simulink model "MARCH_v1_6"  (R2016a)
settings: Solver=FixedStepDiscrete  StartTime=0.0  StopTime=inf  FixedStep=0.001  RelTol=1e-3
InitFcn:
  | cd(fileparts(which(bdroot)));
  | 
  | init_model
  | initialize_model_testingBlocks
StartFcn:
  | cd(fileparts(which(bdroot)));
StopFcn:
  | cd(fileparts(which(bdroot)));
model workspace (MAT data in the model file):
  localValue = 1
  targetValue = 1
undefined symbols (not defined in the file or in its folder): Hip_HAA, Left_Leg, Right_Leg
libraries: xpcethercatlib x56, slrtlib x8, simulink x1, dspnetwork x1, aerolibanimutils x1
(part 1 of 2)
CloseFcn:
  | cd(fileparts(which(bdroot)));
settings Model: SimulationMode=external  Creator=Projectmarch  LastModifiedBy=Projectmarch
settings SolverCC: EnableConcurrentExecution=on
settings DataIOCC: SaveFormat=StructureWithTime
settings OptimizationCC: BlockReduction=off  OptimizeBlockIOStorage=off  BufferReuse=off  GlobalBufferReuse=off  ExpressionFolding=off  LocalBlockOutputs=off
settings HardwareCC: ProdBitPerPointer=32  ProdLargestAtomicFloat=None  ProdWordSize=32  ProdLongLongMode=on  ProdHWDeviceType=Generic->32-bit x86 compatible
settings RTWCC: SystemTargetFile=slrt.tlc  TemplateMakefile=slrt_default_tmf  Description=Simulink Real-Time

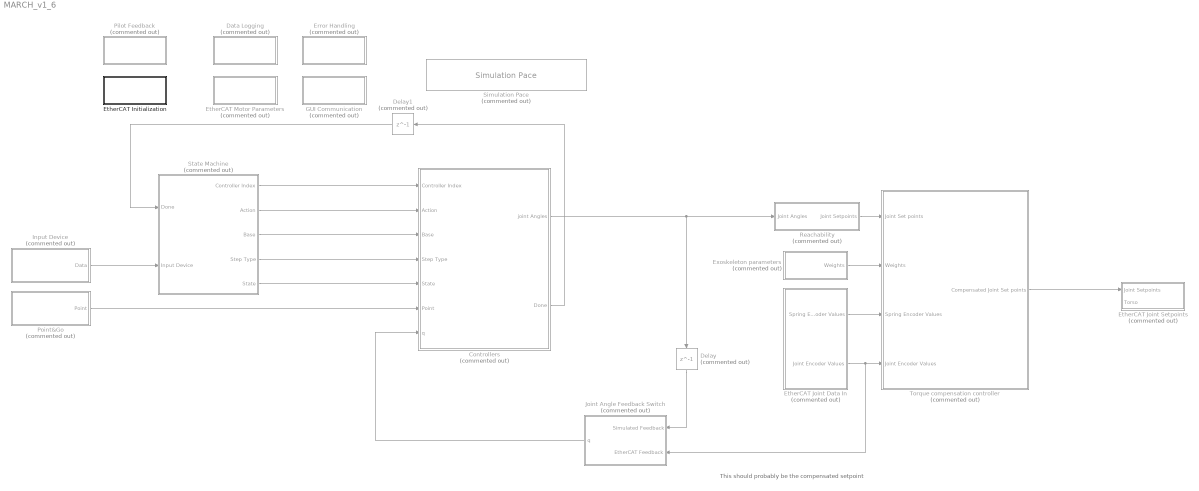
== system MARCH_v1_6 ==
  note: This should probably be the compensated setpoint
  Controllers : Subsystem  Commented=on
  Data Logging : Subsystem  Commented=on
  Delay : Delay  Commented=on  DelayLength=1
  Delay1 : Delay  Commented=on  DelayLength=1
  Error Handling : Subsystem  Commented=on
  EtherCAT Initialization : Subsystem
  EtherCAT Joint Data In : Subsystem  Commented=on
  EtherCAT Joint Setpoints : Subsystem  Commented=on
  EtherCAT Motor Parameters : Subsystem  Commented=on
  Exoskeleton parameters : Subsystem  Commented=on
  GUI Communication : Subsystem  Commented=on
  Input Device : Subsystem  Commented=on
  Joint Angle Feedback Switch : Subsystem  Commented=on
  Pilot Feedback : Subsystem  Commented=on
  Point&Go : Subsystem  Commented=on
  Reachability : Subsystem  Commented=on
  Simulation Pace : aerolibanimutils/Simulation Pace  Commented=on  SimulationPace=1  SleepMode=MATLAB Thread  OutputPaceError=off  SampleTime=-1
  State Machine : Subsystem  Commented=on
  Torque compensation controller : Subsystem  Commented=on
  wires:
  Torque compensation controller/1(Compensated Joint Set points) -> EtherCAT Joint Setpoints/1(Joint Setpoints)
  Reachability/1(Joint Setpoints) -> Torque compensation controller/1(Joint Set points)
  EtherCAT Joint Data In/1(Spring Encoder Values) -> Torque compensation controller/3(Spring Encoder Values)
  EtherCAT Joint Data In/2(Joint Encoder Values) -> Joint Angle Feedback Switch/2(EtherCAT Feedback), Torque compensation controller/4(Joint Encoder Values)
  Exoskeleton parameters/1(Weights) -> Torque compensation controller/2(Weights)
  Controllers/1(joint Angles) -> Reachability/1(Joint Angles), Delay/1
  Delay/1 -> Joint Angle Feedback Switch/1(Simulated Feedback)
  Point&Go/1(Point) -> Controllers/6(Point)
  Input Device/1(Data) -> State Machine/2(Input Device)
  Controllers/2(Done) -> Delay1/1
  State Machine/4(Step Type) -> Controllers/4(Step Type)
  State Machine/2(Action) -> Controllers/2(Action)
  State Machine/3(Base) -> Controllers/3(Base)
  State Machine/1(Controller Index) -> Controllers/1(Controller Index)
  State Machine/5(State) -> Controllers/5(State)
  Joint Angle Feedback Switch/1(q) -> Controllers/7(q)
  Delay1/1 -> State Machine/1(Done)

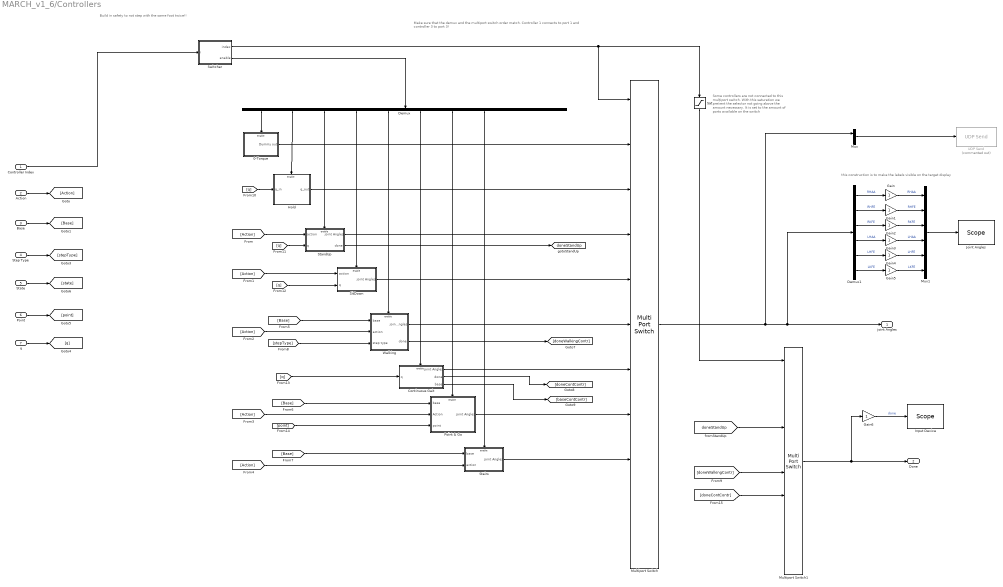
== system MARCH_v1_6/Controllers ==
  note: Some controllers are not connected to this multiport switch. With this saturation we prevent the selector not going above the amount necessary. It is set to the amount of ports available on the switch
  note: Build in safety to not step with the same
      | foot twice!!
  note: Make sure that the demux and the multiport switch order match.
      | Controller 1 connects to port 1 and controller 3 to port 3!
  note: this construction is to make the labels visible on the target display
  Controller Index : Inport
  Action : Inport  Port=2
  Base : Inport  Port=3
  Step Type : Inport  Port=4
  State : Inport  Port=5
  Point : Inport  Port=6
  q : Inport  Port=7
  0-Torque : Subsystem
  Continuous Gait : Subsystem
  Demux : Demux  Outputs=10
  Demux1 : Demux  Outputs=6
  Gain{,1..6} (7 alike) : Gain
  Hold : Subsystem
  "Input Device " : slrtlib/Displays and Logging/Scope   scopeno=4  scopetype=Target  autostart=on  viewmode=Graphical sliding  formatstr='%15.6f'  grid=on  ylimits=[0,0]  nosamples=25000  noprepostsamples=0  interleave=1  triggermode=FreeRun  triggersignal=1  trigsignalfromport=off  triggerlevel=0.0  triggerslope=Either  triggerscope=1  triggersample=0  filename=data.dat  mode=Lazy  writesize=512  autorestart=off  dynamicfilemode=off  maxwritefilesize=512*1024^2
  Joint Angles : slrtlib/Displays and Logging/Scope   scopeno=3  scopetype=Target  autostart=on  viewmode=Graphical sliding  formatstr='%15.6f'  grid=on  ylimits=[0,0]  nosamples=25000  noprepostsamples=0  interleave=1  triggermode=FreeRun  triggersignal=1  trigsignalfromport=off  triggerlevel=0.0  triggerslope=Either  triggerscope=1  triggersample=0  filename=data.dat  mode=Lazy  writesize=512  autorestart=off  dynamicfilemode=off  maxwritefilesize=512*1024^2
  Multiport Switch : MultiPortSwitch  Inputs=10
  Multiport Switch1 : MultiPortSwitch  Inputs=8  DataPortForDefault=Additional data port
  Mux : Mux  Inputs=2
  Mux1 : Mux  Inputs=6
  Point & Go : Subsystem
  Saturation : Saturate  UpperLimit=8  LowerLimit=1
  SitDown : Subsystem
  Stairs : Subsystem
  StandUp : Subsystem
  Switcher : MATLAB Function  TreatAsAtomicUnit=on
  UDP Send : dspnetwork/UDP Send  Commented=on  remoteURL='127.0.0.1'  remotePort=25000  localURL='0.0.0.0'  localPortSource=Automatically determine  localPort=-1  sampletime=-1  separateLengthPort=0
  Walking : Subsystem
  joint Angles : Outport
  Done : Outport  Port=2
  tag scope: doneStandUp=global
  wires:
  Controller Index/1 -> Switcher/1(i)
  Switcher/1(index) -> Saturation/1, Multiport Switch/1
  Switcher/2(enable) -> Demux/1
  Multiport Switch1/1 -> Gain6/1, Done/1
  Mux/1 -> UDP Send/1
  Saturation/1 -> Multiport Switch1/1
  Demux/1 -> 0-Torque/Enable
  Demux/2 -> Hold/Enable
  Demux/3 -> StandUp/Enable
  Demux/4 -> SitDown/Enable
  Demux/5 -> Walking/Enable
  Demux/6 -> Continuous Gait/Enable
  Demux/7 -> Point & Go/Enable
  Demux/8 -> Stairs/Enable
  0-Torque/1(Dummy out) -> Multiport Switch/2
  Hold/1(q_out) -> Multiport Switch/3
  StandUp/1(joint Angles) -> Multiport Switch/4
  SitDown/1(joint Angles) -> Multiport Switch/5
  Walking/1(joint Angles) -> Multiport Switch/6
  Point & Go/1(joint Angles) -> Multiport Switch/8
  Stairs/1(joint Angles) -> Multiport Switch/9
  Action/1 -> [Action]
  Base/1 -> [Base]
  Point/1 -> [point]
  q/1 -> [q]
  Step Type/1 -> [stepType]
  [Action] -> StandUp/1(action)
  [Action] -> SitDown/1(action)
  [Action] -> Walking/2(action)
  [Action] -> Point & Go/2(Action)
  [Action] -> Stairs/2(action)
  [Base] -> Walking/1(base)
  [Base] -> Point & Go/1(base)
  [Base] -> Stairs/1(base)
  [stepType] -> Walking/3(step type)
  [q] -> Hold/1(q_in)
  [q] -> StandUp/2("q ")
  [q] -> SitDown/2("q ")
  [q] -> Continuous Gait/1(q)
  [point] -> Point & Go/3(point)
  Walking/2(done) -> [doneWalkingContr]
  Continuous Gait/2(done) -> [doneContContr]
  Continuous Gait/3(base) -> [baseContContr]
  [doneWalkingContr] -> Multiport Switch1/6
  [doneContContr] -> Multiport Switch1/7
  State/1 -> [state]
  Continuous Gait/1(joint Angles) -> Multiport Switch/7
  StandUp/2(done) -> [doneStandUp]
  [doneStandUp] -> Multiport Switch1/4
  Multiport Switch/1 -> Mux/1, joint Angles/1, Demux1/1
  Demux1/1 -> Gain/1  "RHAA"
  Demux1/2 -> Gain1/1  "RHFE"
  Demux1/3 -> Gain2/1  "RKFE"
  Demux1/4 -> Gain3/1  "LHAA"
  Demux1/5 -> Gain4/1  "LHFE"
  Demux1/6 -> Gain5/1  "LKFE"
  Mux1/1 -> Joint Angles/1
  Gain/1 -> Mux1/1  "RHAA"
  Gain1/1 -> Mux1/2  "RHFE"
  Gain2/1 -> Mux1/3  "RKFE"
  Gain3/1 -> Mux1/4  "LHAA"
  Gain4/1 -> Mux1/5  "LHFE"
  Gain5/1 -> Mux1/6  "LKFE"
  Gain6/1 -> "Input Device "/1  "done"

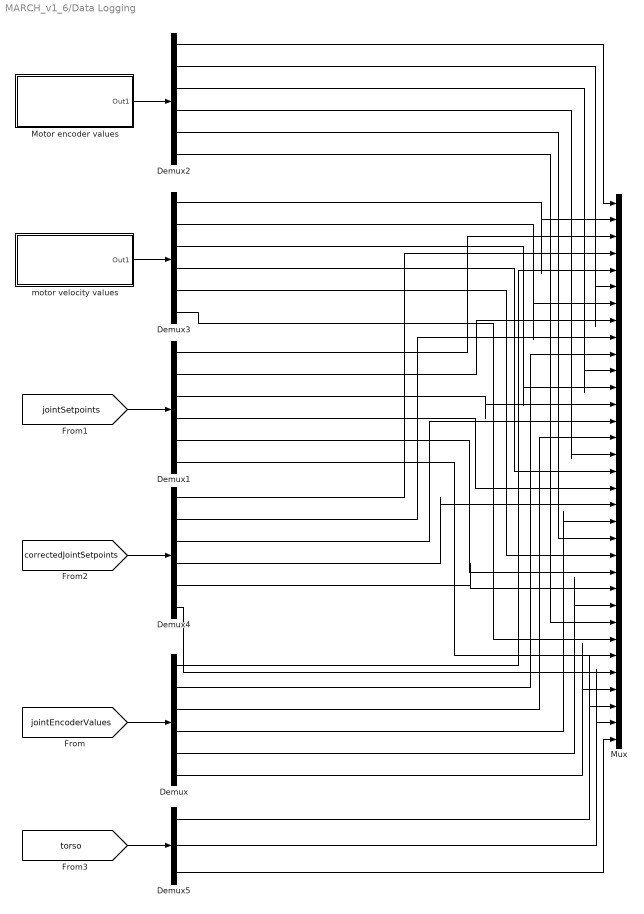
== system MARCH_v1_6/Data Logging ==
  Demux{,1..4} (5 alike) : Demux  Outputs=6
  Demux5 : Demux  Outputs=3
  Motor encoder values : Subsystem
  Mux : Mux  Inputs=33
  motor velocity values : Subsystem
  wires:
  [jointEncoderValues] -> Demux/1
  [jointSetpoints] -> Demux1/1
  Motor encoder values/1(Out1) -> Demux2/1
  motor velocity values/1(Out1) -> Demux3/1
  Demux2/1 -> Mux/1
  Demux3/1 -> Mux/2
  [correctedJointSetpoints] -> Demux4/1
  [torso] -> Demux5/1
  Demux1/1 -> Mux/3
  Demux4/1 -> Mux/4
  Demux/1 -> Mux/5
  Demux2/2 -> Mux/6
  Demux3/2 -> Mux/7
  Demux1/2 -> Mux/8
  Demux4/2 -> Mux/9
  Demux/2 -> Mux/10
  Demux2/3 -> Mux/11
  Demux3/3 -> Mux/12
  Demux1/3 -> Mux/13
  Demux4/3 -> Mux/14
  Demux/3 -> Mux/15
  Demux2/4 -> Mux/16
  Demux2/6 -> Mux/26
  Demux3/4 -> Mux/17
  Demux1/4 -> Mux/18
  Demux4/4 -> Mux/19
  Demux/4 -> Mux/20
  Demux2/5 -> Mux/21
  Demux3/5 -> Mux/22
  Demux1/5 -> Mux/23
  Demux4/5 -> Mux/24
  Demux/5 -> Mux/25
  Demux3/6 -> Mux/27
  Demux1/6 -> Mux/28
  Demux5/3 -> Mux/33
  Demux5/2 -> Mux/32
  Demux5/1 -> Mux/31
  Demux/6 -> Mux/30
  Demux4/6 -> Mux/29

== system MARCH_v1_6/Error Handling ==

== system MARCH_v1_6/EtherCAT Initialization ==
  EtherCAT Init : xpcethercatlib/EtherCAT Init   Priority=0  config_file=D:\Software\MATLAB\simulink-models\EtherCAT Config files\full_setup_v1.0.xml  device_id=0  pci_bus=2  pci_slot=0  dctuning=1  enaDebug=off  enaDC=on  errLink=on  masterDbg=on  stateChgDbg=on  baseClock=off  masterCfg=off  logFile='c:\dbglog.txt'  sample_time=0.001000
  Terminator : Terminator
  wires:
  EtherCAT Init/1 -> Terminator/1

== system MARCH_v1_6/EtherCAT Joint Data In ==
  Data Type Conversion : DataTypeConversion  OutDataTypeStr=double
  Joint Encoder EtherCAT : Subsystem
  MATLAB Function : MATLAB Function  TreatAsAtomicUnit=on
  Spring Encoder EtherCAT : Subsystem
  Spring Encoder Values : Outport
  Joint Encoder Values : Outport  Port=2
  tag scope: jointEncoderValues=global
  wires:
  Spring Encoder EtherCAT/1(Spring Encoder Values) -> Spring Encoder Values/1
  Joint Encoder EtherCAT/1(Joint Encoder Values) -> Data Type Conversion/1, [jointEncoderValues]
  MATLAB Function/1(angles) -> Joint Encoder Values/1
  Data Type Conversion/1 -> MATLAB Function/1(encoderValue)

== system MARCH_v1_6/EtherCAT Joint Setpoints ==
  Joint Setpoints : Inport
  Torso : Inport  Port=2
  Subsystem : Subsystem
  exoskeleton : Subsystem
  wires:
  Joint Setpoints/1 -> exoskeleton/1(Joint setpoints), Subsystem/1(Joint Setpoints)
  Torso/1 -> Subsystem/2(Torso)

== system MARCH_v1_6/EtherCAT Motor Parameters ==
  Hips : Subsystem
  Left Leg : Subsystem
  Right Leg : Subsystem

== system MARCH_v1_6/Exoskeleton parameters ==
  Constant : Constant
  Weights : Outport
  wires:
  Constant/1 -> Weights/1

== system MARCH_v1_6/GUI Communication ==

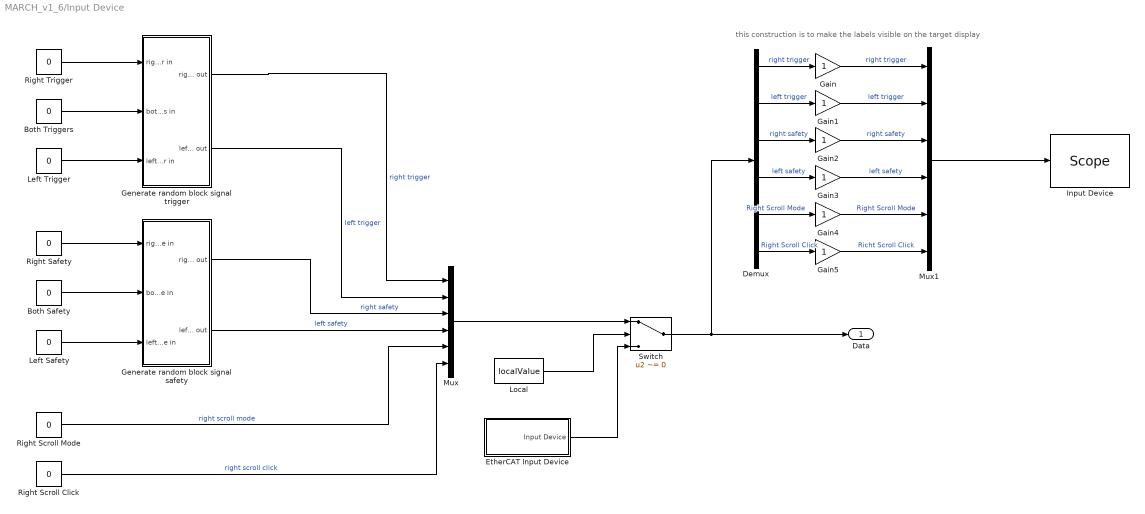
== system MARCH_v1_6/Input Device ==
  note: this construction is to make the labels visible on the target display
  Both Safety : Constant  Value=0
  Both Triggers : Constant  Value=0
  Demux : Demux  Outputs=6
  EtherCAT Input Device : Subsystem
  Gain{,1..5} (6 alike) : Gain
  Generate random block signal safety : Subsystem
  Generate random block signal trigger : Subsystem
  "Input Device " : slrtlib/Displays and Logging/Scope   scopeno=1  scopetype=Target  autostart=on  viewmode=Numerical  formatstr='%15.6f'  grid=on  ylimits=[0,0]  nosamples=25  noprepostsamples=0  interleave=1  triggermode=FreeRun  triggersignal=1  trigsignalfromport=off  triggerlevel=0.0  triggerslope=Either  triggerscope=1  triggersample=0  filename=data.dat  mode=Lazy  writesize=512  autorestart=off  dynamicfilemode=off  maxwritefilesize=512*1024^2
  Left Safety : Constant  Value=0
  Left Trigger : Constant  Value=0
  Local : Constant  Value=localValue
  Mux : Mux  Inputs=6
  Mux1 : Mux  Inputs=6
  Right Safety : Constant  Value=0
  Right Scroll Click : Constant  Value=0
  Right Scroll Mode : Constant  Value=0
  Right Trigger : Constant  Value=0
  Switch : Switch  Criteria=u2 ~= 0
  Data : Outport
  wires:
  Mux/1 -> Switch/1
  Switch/1 -> Demux/1, Data/1
  Local/1 -> Switch/2
  EtherCAT Input Device/1(Input Device) -> Switch/3
  Right Scroll Mode/1 -> Mux/5  "right scroll mode"
  Right Safety/1 -> Generate random block signal safety/1(right safe in)
  Right Scroll Click/1 -> Mux/6  "right scroll click"
  Right Trigger/1 -> Generate random block signal trigger/1(rightTrigger in)
  Left Trigger/1 -> Generate random block signal trigger/3("leftTrigger in ")
  Both Triggers/1 -> Generate random block signal trigger/2(bothTriggers in)
  Generate random block signal trigger/1(rightTrigger out) -> Mux/1  "right trigger"
  Generate random block signal trigger/2(leftTrigger out) -> Mux/2  "left trigger"
  Generate random block signal safety/1(right safe out) -> Mux/3  "right safety"
  Generate random block signal safety/2(left safe out) -> Mux/4  "left safety"
  Left Safety/1 -> Generate random block signal safety/3("left safe in ")
  Both Safety/1 -> Generate random block signal safety/2(both safe in)
  Mux1/1 -> "Input Device "/1
  Demux/1 -> Gain/1  "right trigger"
  Demux/2 -> Gain1/1  "left trigger"
  Demux/3 -> Gain2/1  "right safety"
  Demux/4 -> Gain3/1  "left safety"
  Demux/5 -> Gain4/1  "Right Scroll Mode"
  Demux/6 -> Gain5/1  "Right Scroll Click"
  Gain/1 -> Mux1/1  "right trigger"
  Gain1/1 -> Mux1/2  "left trigger"
  Gain2/1 -> Mux1/3  "right safety"
  Gain3/1 -> Mux1/4  "left safety"
  Gain4/1 -> Mux1/5  "Right Scroll Mode"
  Gain5/1 -> Mux1/6  "Richt Scroll Click"

== system MARCH_v1_6/Joint Angle Feedback Switch ==
  Simulated Feedback : Inport
  EtherCAT Feedback : Inport  Port=2
  Local : Constant  Value=0
  Switch : Switch  Criteria=u2 ~= 0
  q : Outport
  wires:
  EtherCAT Feedback/1 -> Switch/3
  Switch/1 -> q/1
  Simulated Feedback/1 -> Switch/1
  Local/1 -> Switch/2

== system MARCH_v1_6/Pilot Feedback ==

== system MARCH_v1_6/Point&Go ==
  note: For now, always use dummy point and go data even during target runs
  EtherCAT Point&Go : Subsystem
  Local : Constant  Value=localValue
  Point & Go Point : Constant  Value=[0.1 -0.3 0]
  Switch : Switch  Criteria=u2 ~= 0
  Point : Outport
  wires:
  EtherCAT Point&Go/1(Point&Go Data) -> Switch/3
  Local/1 -> Switch/2
  Switch/1 -> Point/1
  Point & Go Point/1 -> Switch/1

== system MARCH_v1_6/Reachability ==
  Joint Angles : Inport
  Data Type Conversion : DataTypeConversion  OutDataTypeStr=uint32
  MATLAB Function : MATLAB Function  Commented=on  TreatAsAtomicUnit=on
  Terminator2 : Terminator  Commented=on
  Joint Setpoints : Outport
  tag scope: jointSetpoints=global
  wires:
  MATLAB Function/2(err) -> Terminator2/1
  Data Type Conversion/1 -> [jointSetpoints]
  Joint Angles/1 -> Data Type Conversion/1, Joint Setpoints/1

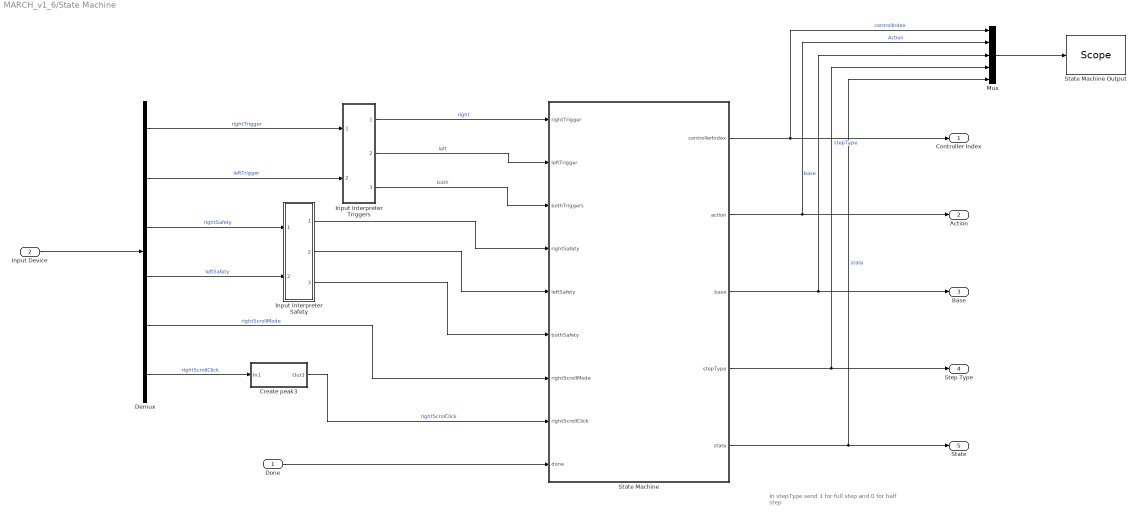
== system MARCH_v1_6/State Machine ==
  note: In stepType send 1 for full step and 0 for half step
  Done : Inport
  Input Device : Inport  Port=2
  Create peak3 : Subsystem
  Demux : Demux  Outputs=6
  Input Interpreter Safety : MATLAB Function  TreatAsAtomicUnit=on
  Input Interpreter Triggers : MATLAB Function  TreatAsAtomicUnit=on
  Mux : Mux  Inputs=5
  State Machine : Stateflow chart  TreatAsAtomicUnit=on
  "State Machine Output " : slrtlib/Displays and Logging/Scope   scopeno=2  scopetype=Target  autostart=on  viewmode=Numerical  formatstr='%15.6f'  grid=on  ylimits=[0,0]  nosamples=25  noprepostsamples=0  interleave=1  triggermode=FreeRun  triggersignal=1  trigsignalfromport=off  triggerlevel=0.0  triggerslope=Either  triggerscope=1  triggersample=0  filename=data.dat  mode=Lazy  writesize=512  autorestart=off  dynamicfilemode=off  maxwritefilesize=512*1024^2
  Controller Index : Outport
  Action : Outport  Port=2
  Base : Outport  Port=3
  Step Type : Outport  Port=4
  State : Outport  Port=5
  wires:
  Demux/2 -> Input Interpreter Triggers/2(leftIn)  "leftTrigger"
  Demux/3 -> Input Interpreter Safety/1(rightIn)  "rightSafety"
  Demux/4 -> Input Interpreter Safety/2(leftIn)  "leftSafety"
  Demux/5 -> State Machine/7(rightScrollMode)  "rightScrollMode"
  Demux/6 -> Create peak3/1(In1)  "rightScrollClick"
  Demux/1 -> Input Interpreter Triggers/1(rightIn)  "rightTrigger"
  Input Interpreter Triggers/1(rightOut) -> State Machine/1(rightTrigger)  "right"
  Input Interpreter Triggers/2(leftOut) -> State Machine/2(leftTrigger)  "left"
  Input Interpreter Triggers/3(bothOut) -> State Machine/3(bothTriggers)  "both"
  Input Interpreter Safety/2(leftOut) -> State Machine/5(leftSafety)
  Input Interpreter Safety/3(bothOut) -> State Machine/6(bothSafety)
  Create peak3/1(Out1) -> State Machine/8(rightScrollClick)  "rightScrolClick"
  Input Interpreter Safety/1(rightOut) -> State Machine/4(rightSafety)
  Input Device/1 -> Demux/1
  Done/1 -> State Machine/9(done)
  State Machine/5(state) -> Mux/5, State/1  "state"
  State Machine/1(controllerIndex) -> Mux/1, Controller Index/1  "controlIndex"
  State Machine/2(action) -> Mux/2, Action/1  "Action"
  State Machine/3(base) -> Mux/3, Base/1  "base"
  State Machine/4(stepType) -> Mux/4, Step Type/1  "stepType"
  Mux/1 -> "State Machine Output "/1

== system MARCH_v1_6/Torque compensation controller ==
  Joint Set points : Inport
  Weights : Inport  Port=2
  Spring Encoder Values : Inport  Port=3
  Joint Encoder Values : Inport  Port=4
  Terminator : Terminator
  Terminator1 : Terminator
  Terminator2 : Terminator
  Compensated Joint Set points : Outport
  wires:
  Joint Set points/1 -> Compensated Joint Set points/1
  Joint Encoder Values/1 -> Terminator2/1
  Spring Encoder Values/1 -> Terminator1/1
  Weights/1 -> Terminator/1

== system MARCH_v1_6/Controllers/0-Torque ==
  note: Since we don't control joint angles but motor velocity we just send dummy joint angles instead. This is a 1x6 vector of zeros.
  Enable : EnablePort  StatesWhenEnabling=reset
  Constant : Constant  Value=[0 0 0 0 0 0 ]
  RHFE : Subsystem
  Dummy out : Outport  InitialOutput=[0 0 0 0 0 0]
  wires:
  Constant/1 -> Dummy out/1

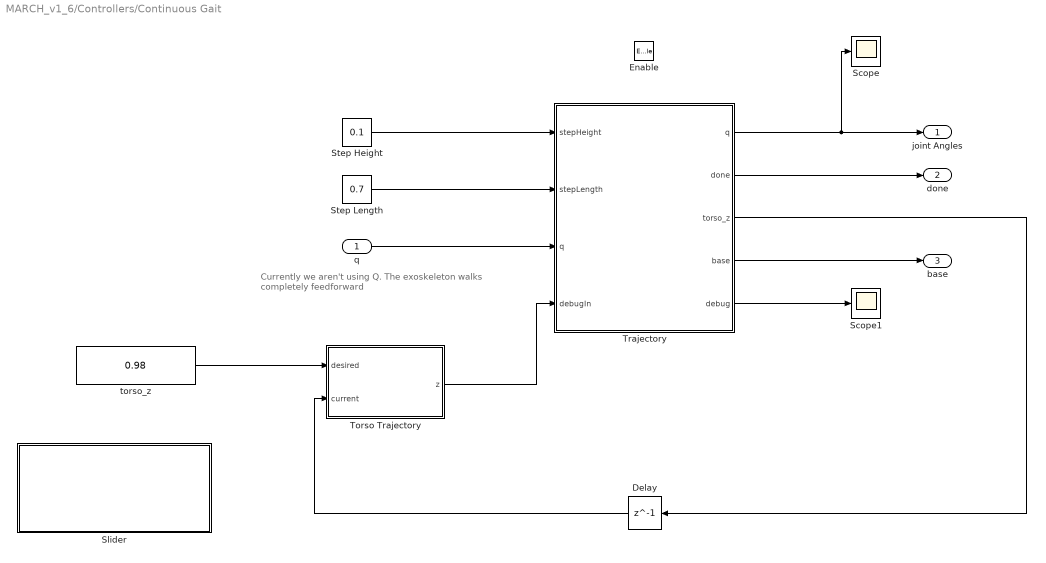
== system MARCH_v1_6/Controllers/Continuous Gait ==
  note: Currently we aren't using Q. The exoskeleton walks completely feedforward
  q : Inport
  Enable : EnablePort  StatesWhenEnabling=reset
  Delay : Delay  DelayLength=1  InitialCondition=1
  Scope : Scope
  Scope1 : Scope
  Slider : Subsystem  DialogController=hmiCreateDDGDialog  IsWebBlock=on  mask(MWDashboardBlock){webBlockId=08960381-2fc9-439b-949a-5d55ec4678c5, webBlockType=slider, ShowInLibBrowser=on, ShowInitialText=on, HMISrcModelName=MARCH_v1_6}
      mask prompts: webBlockId "WebBlock Id"; webBlockType "WebBlock Type"; HMISrcModelName "Source Model"
      mask Help: helpview([docroot '/mapfiles/simulink.map'], 'hmi_slider')
      mask Display:
      | if strcmp(get_param(bdroot(gcb),'BlockDiagramType'), 'library')
      |     image([(matlabroot) '/toolbox/simulink/hmi/icons/Slider.png']);
      | end
  Step Height : Constant  Value=0.1
  Step Length : Constant  Value=0.7
  Torso Trajectory : MATLAB Function  TreatAsAtomicUnit=on
  Trajectory : MATLAB Function  TreatAsAtomicUnit=on
  torso_z : Constant  Value=0.98
  joint Angles : Outport
  done : Outport  Port=2
  base : Outport  Port=3
  wires:
  Step Length/1 -> Trajectory/2(stepLength)
  Trajectory/1(q) -> Scope/1, joint Angles/1
  q/1 -> Trajectory/3("q ")
  Step Height/1 -> Trajectory/1(stepHeight)
  Trajectory/3(torso_z) -> Delay/1
  torso_z/1 -> Torso Trajectory/1(desired)
  Torso Trajectory/1(z) -> Trajectory/4(debugIn)
  Delay/1 -> Torso Trajectory/2(current)
  Trajectory/4(base) -> base/1
  Trajectory/2(done) -> done/1
  Trajectory/5(debug) -> Scope1/1

== system MARCH_v1_6/Controllers/Hold ==
  q_in : Inport
  Enable : EnablePort
  Constant : Constant  Value=0
  MATLAB Function : MATLAB Function  TreatAsAtomicUnit=on
  q_out : Outport
  wires:
  q_in/1 -> MATLAB Function/1(q_in)
  MATLAB Function/1(q_out) -> q_out/1
  Constant/1 -> MATLAB Function/2(reset)

== system MARCH_v1_6/Controllers/Point & Go ==
  base : Inport
  Action : Inport  Port=2
  point : Inport  Port=3
  Enable : EnablePort  StatesWhenEnabling=reset
  Scope : Scope
  Scope1 : Scope
  Trajectory : MATLAB Function  TreatAsAtomicUnit=on
  "stop " : Constant  Value=0
  joint Angles : Outport
  wires:
  Trajectory/1(q) -> Scope/1, joint Angles/1
  Action/1 -> Trajectory/2(action)
  Trajectory/2(debugOut) -> Scope1/1
  base/1 -> Trajectory/1(base)
  point/1 -> Trajectory/3(point)
  "stop "/1 -> Trajectory/5(debugIn)

== system MARCH_v1_6/Controllers/SitDown ==
  action : Inport
  "q " : Inport  Port=2
  Enable : EnablePort  StatesWhenEnabling=reset
  Constant : Constant  Value=[0 -1.92 1.8 0 -1.92 1.8]
  Trajectory : MATLAB Function  TreatAsAtomicUnit=on
  joint Angles : Outport
  wires:
  Trajectory/1(q) -> joint Angles/1
  action/1 -> Trajectory/1(action)
  Constant/1 -> Trajectory/2(q_i)

== system MARCH_v1_6/Controllers/Stairs ==
  note: Only use positive values for this y-element. The trajectory block takes care which side to shift the weight to based on the swing foot
  base : Inport
  action : Inport  Port=2
  Enable : EnablePort  StatesWhenEnabling=reset
  Scope : Scope  NumInputPorts=2
  Torso Trajectory : MATLAB Function  Commented=on  TreatAsAtomicUnit=on
  Trajectory : MATLAB Function  TreatAsAtomicUnit=on
  action c : Constant
  base c : Constant  Value=3
  torso_delta : Constant  Value=[0, 0.1, 0.00]
  joint Angles : Outport
  wires:
  Trajectory/1(q) -> Scope/1, joint Angles/1
  action c/1 -> Trajectory/2(action_t)
  base c/1 -> Trajectory/1(base)
  torso_delta/1 -> Trajectory/4(torso_delta)

== system MARCH_v1_6/Controllers/StandUp ==
  note: These are the Q values when the exoskeleton is seated with the torso fully tilted forward
  action : Inport
  "q " : Inport  Port=2
  Enable : EnablePort  StatesWhenEnabling=reset
  Simulation Q : Constant  Value=[0 -1.92 1.8 0 -1.92 1.8]
  Trajectory : MATLAB Function  TreatAsAtomicUnit=on
  joint Angles : Outport
  done : Outport  Port=2
  wires:
  Trajectory/2(q) -> joint Angles/1
  action/1 -> Trajectory/1(action)
  "q "/1 -> Trajectory/2(q_i)
  Trajectory/1(done) -> done/1

== system MARCH_v1_6/Controllers/Walking ==
  base : Inport
  action : Inport  Port=2
  step type : Inport  Port=3
  Enable : EnablePort  StatesWhenEnabling=reset
  Mux : Mux  Inputs=3
  Trajectory : MATLAB Function  TreatAsAtomicUnit=on
  joint Angles : Outport
  done : Outport  Port=2
  wires:
  Trajectory/1(q) -> joint Angles/1
  action/1 -> Mux/2, Trajectory/2(action)  "action"
  base/1 -> Mux/1, Trajectory/1(base)  "base"
  Trajectory/2(done) -> done/1
  step type/1 -> Mux/3, Trajectory/3(stepType)  "step type"

== system MARCH_v1_6/Data Logging/Motor encoder values ==
  Data Type Conversion : DataTypeConversion  OutDataTypeStr=uint32
  EtherCAT PDO Receive1 : xpcethercatlib/EtherCAT PDO Receive  Priority=2  sig_name=RHFE.Inputs.motorAngle  sig_offset=12528  sig_type=uint16  type_size=16  sig_dim=1  device_id=0  sample_time=0.001000
  EtherCAT PDO Receive2 : xpcethercatlib/EtherCAT PDO Receive  Priority=2  sig_name=RHFE.Inputs.motorAngle  sig_offset=12528  sig_type=uint16  type_size=16  sig_dim=1  device_id=0  sample_time=0.001000
  EtherCAT PDO Receive3 : xpcethercatlib/EtherCAT PDO Receive  Priority=2  sig_name=LHFE.Inputs.motorAngle  sig_offset=240  sig_type=uint16  type_size=16  sig_dim=1  device_id=0  sample_time=0.001000
  EtherCAT PDO Receive4 : xpcethercatlib/EtherCAT PDO Receive  Priority=2  sig_name=LHFE.Inputs.motorAngle  sig_offset=240  sig_type=uint16  type_size=16  sig_dim=1  device_id=0  sample_time=0.001000
  EtherCAT PDO Receive5 : xpcethercatlib/EtherCAT PDO Receive  Priority=2  sig_name=RKFE.Inputs.motorAngle  sig_offset=12816  sig_type=uint16  type_size=16  sig_dim=1  device_id=0  sample_time=0.001000
  EtherCAT PDO Receive7 : xpcethercatlib/EtherCAT PDO Receive  Priority=2  sig_name=LKFE.Inputs.motorAngle  sig_offset=528  sig_type=uint16  type_size=16  sig_dim=1  device_id=0  sample_time=0.001000
  Mux1 : Mux  Inputs=6
  Out1 : Outport
  wires:
  EtherCAT PDO Receive4/1 -> Mux1/4
  EtherCAT PDO Receive5/1 -> Mux1/3
  EtherCAT PDO Receive7/1 -> Mux1/6
  Mux1/1 -> Data Type Conversion/1
  EtherCAT PDO Receive1/1 -> Mux1/1
  EtherCAT PDO Receive3/1 -> Mux1/5
  EtherCAT PDO Receive2/1 -> Mux1/2
  Data Type Conversion/1 -> Out1/1

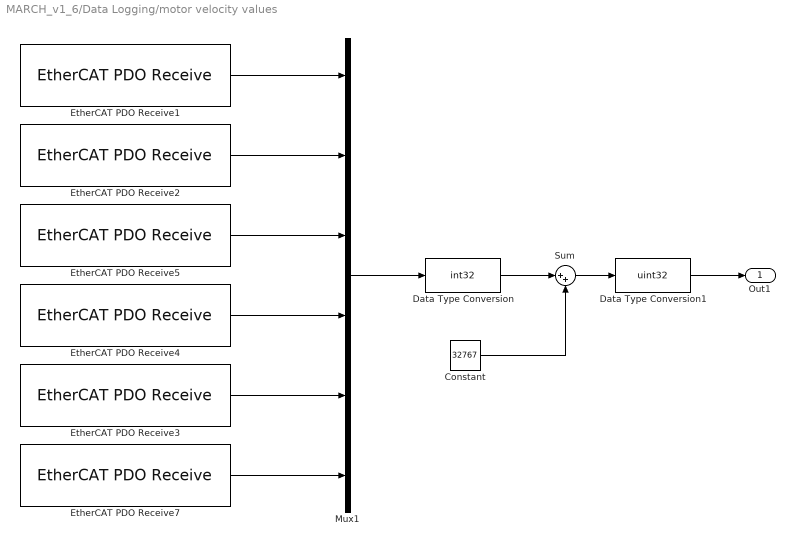
== system MARCH_v1_6/Data Logging/motor velocity values ==
  Constant : Constant  Value=32767
  Data Type Conversion : DataTypeConversion  OutDataTypeStr=int32
  Data Type Conversion1 : DataTypeConversion  OutDataTypeStr=uint32
  EtherCAT PDO Receive1 : xpcethercatlib/EtherCAT PDO Receive  Priority=2  sig_name=RHFE.Inputs.motorVelocity  sig_offset=12544  sig_type=int16  type_size=16  sig_dim=1  device_id=0  sample_time=0.001000
  EtherCAT PDO Receive2 : xpcethercatlib/EtherCAT PDO Receive  Priority=2  sig_name=RHFE.Inputs.motorVelocity  sig_offset=12544  sig_type=int16  type_size=16  sig_dim=1  device_id=0  sample_time=0.001000
  EtherCAT PDO Receive3 : xpcethercatlib/EtherCAT PDO Receive  Priority=2  sig_name=LHFE.Inputs.motorVelocity  sig_offset=256  sig_type=int16  type_size=16  sig_dim=1  device_id=0  sample_time=0.001000
  EtherCAT PDO Receive4 : xpcethercatlib/EtherCAT PDO Receive  Priority=2  sig_name=LHFE.Inputs.motorVelocity  sig_offset=256  sig_type=int16  type_size=16  sig_dim=1  device_id=0  sample_time=0.001000
  EtherCAT PDO Receive5 : xpcethercatlib/EtherCAT PDO Receive  Priority=2  sig_name=RKFE.Inputs.motorVelocity  sig_offset=12832  sig_type=int16  type_size=16  sig_dim=1  device_id=0  sample_time=0.001000
  EtherCAT PDO Receive7 : xpcethercatlib/EtherCAT PDO Receive  Priority=2  sig_name=LKFE.Inputs.motorVelocity  sig_offset=544  sig_type=int16  type_size=16  sig_dim=1  device_id=0  sample_time=0.001000
  Mux1 : Mux  Inputs=6
  Sum : Sum  Inputs=|++
  Out1 : Outport
  wires:
  EtherCAT PDO Receive2/1 -> Mux1/2
  EtherCAT PDO Receive3/1 -> Mux1/5
  EtherCAT PDO Receive1/1 -> Mux1/1
  Mux1/1 -> Data Type Conversion/1
  EtherCAT PDO Receive7/1 -> Mux1/6
  EtherCAT PDO Receive5/1 -> Mux1/3
  EtherCAT PDO Receive4/1 -> Mux1/4
  Constant/1 -> Sum/2
  Data Type Conversion/1 -> Sum/1
  Sum/1 -> Data Type Conversion1/1
  Data Type Conversion1/1 -> Out1/1

== system MARCH_v1_6/EtherCAT Joint Data In/Joint Encoder EtherCAT ==
  EtherCAT PDO Receive10 : xpcethercatlib/EtherCAT PDO Receive  Priority=2  sig_name=Left_Leg.Inputs.H_jointAngle  sig_offset=1144  sig_type=uint32  type_size=32  sig_dim=1  device_id=0  sample_time=0.001000
  EtherCAT PDO Receive11 : xpcethercatlib/EtherCAT PDO Receive  Priority=2  sig_name=Left_Leg.Inputs.K_jointAngle  sig_offset=1312  sig_type=uint32  type_size=32  sig_dim=1  device_id=0  sample_time=0.001000
  EtherCAT PDO Receive6 : xpcethercatlib/EtherCAT PDO Receive  Priority=2  sig_name=Hip_HAA.Inputs.R_jointAngle  sig_offset=688  sig_type=uint32  type_size=32  sig_dim=1  device_id=0  sample_time=0.001000
  EtherCAT PDO Receive7 : xpcethercatlib/EtherCAT PDO Receive  Priority=2  sig_name=Right_Leg.Inputs.K_jointAngle  sig_offset=2000  sig_type=uint32  type_size=32  sig_dim=1  device_id=0  sample_time=0.001000
  EtherCAT PDO Receive8 : xpcethercatlib/EtherCAT PDO Receive  Priority=2  sig_name=Right_Leg.Inputs.H_jointAngle  sig_offset=1832  sig_type=uint32  type_size=32  sig_dim=1  device_id=0  sample_time=0.001000
  EtherCAT PDO Receive9 : xpcethercatlib/EtherCAT PDO Receive  Priority=2  sig_name=Hip_HAA.Inputs.L_jointAngle  sig_offset=208  sig_type=uint32  type_size=32  sig_dim=1  device_id=0  sample_time=0.001000
  Mux1 : Mux  Inputs=6
  Joint Encoder Values : Outport
  wires:
  EtherCAT PDO Receive7/1 -> Mux1/3
  EtherCAT PDO Receive9/1 -> Mux1/4
  EtherCAT PDO Receive8/1 -> Mux1/2
  EtherCAT PDO Receive6/1 -> Mux1/1
  EtherCAT PDO Receive10/1 -> Mux1/5
  EtherCAT PDO Receive11/1 -> Mux1/6
  Mux1/1 -> Joint Encoder Values/1

== system MARCH_v1_6/EtherCAT Joint Data In/Spring Encoder EtherCAT ==
  EtherCAT PDO Receive : xpcethercatlib/EtherCAT PDO Receive  Priority=2  sig_name=Hip_HAA.Inputs.R_springAngle  sig_offset=720  sig_type=uint32  type_size=32  sig_dim=1  device_id=0  sample_time=0.001000
  EtherCAT PDO Receive1 : xpcethercatlib/EtherCAT PDO Receive  Priority=2  sig_name=Right_Leg.Inputs.H_springAngle  sig_offset=1864  sig_type=uint32  type_size=32  sig_dim=1  device_id=0  sample_time=0.001000
  EtherCAT PDO Receive2 : xpcethercatlib/EtherCAT PDO Receive  Priority=2  sig_name=Right_Leg.Inputs.K_springAngle  sig_offset=2032  sig_type=uint32  type_size=32  sig_dim=1  device_id=0  sample_time=0.001000
  EtherCAT PDO Receive3 : xpcethercatlib/EtherCAT PDO Receive  Priority=2  sig_name=Hip_HAA.Inputs.L_springAngle  sig_offset=240  sig_type=uint32  type_size=32  sig_dim=1  device_id=0  sample_time=0.001000
  EtherCAT PDO Receive4 : xpcethercatlib/EtherCAT PDO Receive  Priority=2  sig_name=Left_Leg.Inputs.H_springAngle  sig_offset=1176  sig_type=uint32  type_size=32  sig_dim=1  device_id=0  sample_time=0.001000
  EtherCAT PDO Receive5 : xpcethercatlib/EtherCAT PDO Receive  Priority=2  sig_name=Left_Leg.Inputs.K_springAngle  sig_offset=1344  sig_type=uint32  type_size=32  sig_dim=1  device_id=0  sample_time=0.001000
  Mux : Mux  Inputs=6
  Spring Encoder Values : Outport
  wires:
  EtherCAT PDO Receive2/1 -> Mux/3
  EtherCAT PDO Receive4/1 -> Mux/5
  Mux/1 -> Spring Encoder Values/1
  EtherCAT PDO Receive5/1 -> Mux/6
  EtherCAT PDO Receive1/1 -> Mux/2
  EtherCAT PDO Receive/1 -> Mux/1
  EtherCAT PDO Receive3/1 -> Mux/4

== system MARCH_v1_6/EtherCAT Joint Setpoints/Subsystem ==
  Joint Setpoints : Inport
  Torso : Inport  Port=2
  Data Type Conversion : DataTypeConversion  OutDataTypeStr=uint32
  Data Type Conversion1 : DataTypeConversion  OutDataTypeStr=uint32
  tag scope: correctedJointSetpoints=global, torso=global
  wires:
  Joint Setpoints/1 -> Data Type Conversion/1
  Torso/1 -> Data Type Conversion1/1
  Data Type Conversion/1 -> [correctedJointSetpoints]
  Data Type Conversion1/1 -> [torso]

== system MARCH_v1_6/EtherCAT Joint Setpoints/exoskeleton ==
  Joint setpoints : Inport
  Data Type Conversion : DataTypeConversion  OutDataTypeStr=uint32
  EtherCAT Joint Communication : Subsystem  Commented=on
  MATLAB Function : MATLAB Function  Commented=on  TreatAsAtomicUnit=on
  "Scope " : slrtlib/Displays and Logging/Scope   Commented=on  scopeno=5  scopetype=Target  autostart=on  viewmode=Numerical  formatstr='%15.6f'  grid=on  ylimits=[0,0]  nosamples=3  noprepostsamples=0  interleave=1  triggermode=FreeRun  triggersignal=1  trigsignalfromport=off  triggerlevel=0.0  triggerslope=Either  triggerscope=1  triggersample=0  filename=data.dat  mode=Lazy  writesize=512  autorestart=off  dynamicfilemode=off  maxwritefilesize=512*1024^2
  Scope 1 : slrtlib/Displays and Logging/Scope   Commented=on  scopeno=5  scopetype=Target  autostart=on  viewmode=Graphical sliding  formatstr='%15.6f'  grid=on  ylimits=[0,0]  nosamples=25000  noprepostsamples=0  interleave=1  triggermode=FreeRun  triggersignal=1  trigsignalfromport=off  triggerlevel=0.0  triggerslope=Either  triggerscope=1  triggersample=0  filename=data.dat  mode=Lazy  writesize=512  autorestart=off  dynamicfilemode=off  maxwritefilesize=512*1024^2
  Scope 2 : slrtlib/Displays and Logging/Scope   Commented=on  scopeno=5  scopetype=Target  autostart=on  viewmode=Numerical  formatstr='%15.6f'  grid=on  ylimits=[0,0]  nosamples=3  noprepostsamples=0  interleave=1  triggermode=FreeRun  triggersignal=1  trigsignalfromport=off  triggerlevel=0.0  triggerslope=Either  triggerscope=1  triggersample=0  filename=data.dat  mode=Lazy  writesize=512  autorestart=off  dynamicfilemode=off  maxwritefilesize=512*1024^2
  Scope 3 : slrtlib/Displays and Logging/Scope   Commented=on  scopeno=5  scopetype=Target  autostart=on  viewmode=Graphical sliding  formatstr='%15.6f'  grid=on  ylimits=[0,0]  nosamples=25000  noprepostsamples=0  interleave=1  triggermode=FreeRun  triggersignal=1  trigsignalfromport=off  triggerlevel=0.0  triggerslope=Either  triggerscope=1  triggersample=0  filename=data.dat  mode=Lazy  writesize=512  autorestart=off  dynamicfilemode=off  maxwritefilesize=512*1024^2
  wires:
  Data Type Conversion/1 -> EtherCAT Joint Communication/1(Joint Setpoints)
  Joint setpoints/1 -> Scope 1/1, "Scope "/1, Data Type Conversion/1, Scope 3/1, Scope 2/1

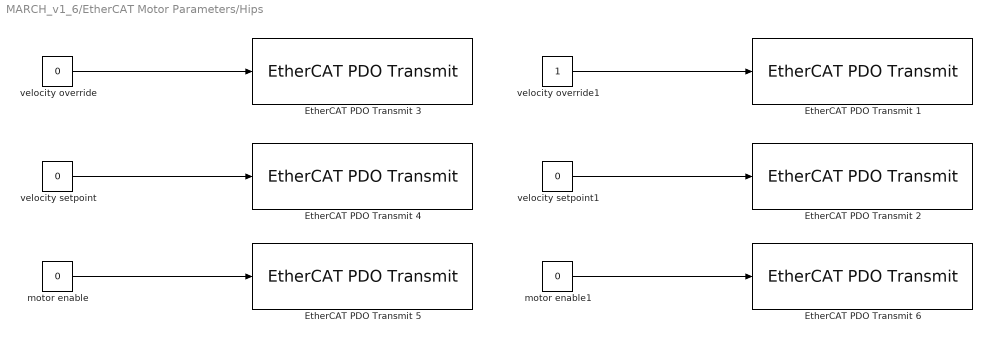
== system MARCH_v1_6/EtherCAT Motor Parameters/Hips ==
  EtherCAT PDO Transmit 1 : xpcethercatlib/EtherCAT PDO Transmit   Priority=3  sig_name=Hip_HAA.Outputs.R_data[4]  sig_offset=784  sig_type=int32  type_size=32  sig_dim=1  device_id=0  sample_time=0.001000
  EtherCAT PDO Transmit 2 : xpcethercatlib/EtherCAT PDO Transmit   Priority=3  sig_name=Hip_HAA.Outputs.R_velocitySetPoint  sig_offset=512  sig_type=int16  type_size=16  sig_dim=1  device_id=0  sample_time=0.001000
  EtherCAT PDO Transmit 3 : xpcethercatlib/EtherCAT PDO Transmit   Priority=3  sig_name=Hip_HAA.Outputs.L_data[4]  sig_offset=480  sig_type=int32  type_size=32  sig_dim=1  device_id=0  sample_time=0.001000
  EtherCAT PDO Transmit 4 : xpcethercatlib/EtherCAT PDO Transmit   Priority=3  sig_name=Hip_HAA.Outputs.L_velocitySetPoint  sig_offset=208  sig_type=int16  type_size=16  sig_dim=1  device_id=0  sample_time=0.001000
  EtherCAT PDO Transmit 5 : xpcethercatlib/EtherCAT PDO Transmit   Priority=3  sig_name=Hip_HAA.Outputs.L_motorEnable  sig_offset=256  sig_type=uint8  type_size=8  sig_dim=1  device_id=0  sample_time=0.001000
  EtherCAT PDO Transmit 6 : xpcethercatlib/EtherCAT PDO Transmit   Priority=3  sig_name=Hip_HAA.Outputs.R_motorEnable  sig_offset=560  sig_type=uint8  type_size=8  sig_dim=1  device_id=0  sample_time=0.001000
  motor enable : Constant  Value=0  OutDataTypeStr=uint8
  motor enable1 : Constant  Value=0  OutDataTypeStr=uint8
  velocity override : Constant  Value=0  OutDataTypeStr=int32
  velocity override1 : Constant  OutDataTypeStr=int32
  velocity setpoint : Constant  Value=0  OutDataTypeStr=int16
  velocity setpoint1 : Constant  Value=0  OutDataTypeStr=int16
  wires:
  motor enable/1 -> EtherCAT PDO Transmit 5/1
  velocity override/1 -> EtherCAT PDO Transmit 3/1
  velocity setpoint/1 -> EtherCAT PDO Transmit 4/1
  motor enable1/1 -> EtherCAT PDO Transmit 6/1
  velocity override1/1 -> EtherCAT PDO Transmit 1/1
  velocity setpoint1/1 -> EtherCAT PDO Transmit 2/1

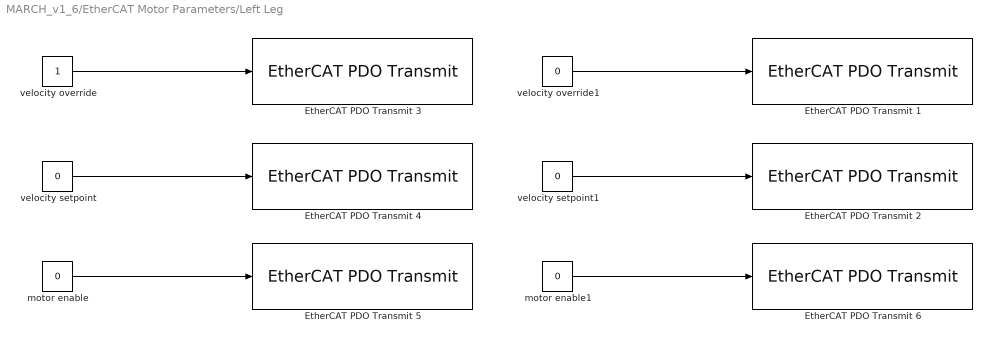
== system MARCH_v1_6/EtherCAT Motor Parameters/Left Leg ==
  EtherCAT PDO Transmit 1 : xpcethercatlib/EtherCAT PDO Transmit   Priority=3  sig_name=Left_Leg.Outputs.K_data[4]  sig_offset=1688  sig_type=int32  type_size=32  sig_dim=1  device_id=0  sample_time=0.001000
  EtherCAT PDO Transmit 2 : xpcethercatlib/EtherCAT PDO Transmit   Priority=3  sig_name=Left_Leg.Outputs.K_velocitySetPoint  sig_offset=1432  sig_type=int16  type_size=16  sig_dim=1  device_id=0  sample_time=0.001000
  EtherCAT PDO Transmit 3 : xpcethercatlib/EtherCAT PDO Transmit   Priority=3  sig_name=Left_Leg.Outputs.H_data[4]  sig_offset=1400  sig_type=int32  type_size=32  sig_dim=1  device_id=0  sample_time=0.001000
  EtherCAT PDO Transmit 4 : xpcethercatlib/EtherCAT PDO Transmit   Priority=3  sig_name=Left_Leg.Outputs.H_velocitySetPoint  sig_offset=1144  sig_type=int16  type_size=16  sig_dim=1  device_id=0  sample_time=0.001000
  EtherCAT PDO Transmit 5 : xpcethercatlib/EtherCAT PDO Transmit   Priority=3  sig_name=Left_Leg.Outputs.H_motorEnable  sig_offset=1192  sig_type=uint8  type_size=8  sig_dim=1  device_id=0  sample_time=0.001000
  EtherCAT PDO Transmit 6 : xpcethercatlib/EtherCAT PDO Transmit   Priority=3  sig_name=Left_Leg.Outputs.K_motorEnable  sig_offset=1480  sig_type=uint8  type_size=8  sig_dim=1  device_id=0  sample_time=0.001000
  motor enable : Constant  Value=0  OutDataTypeStr=uint8
  motor enable1 : Constant  Value=0  OutDataTypeStr=uint8
  velocity override : Constant  OutDataTypeStr=int32
  velocity override1 : Constant  Value=0  OutDataTypeStr=int32
  velocity setpoint : Constant  Value=0  OutDataTypeStr=int16
  velocity setpoint1 : Constant  Value=0  OutDataTypeStr=int16
  wires:
  motor enable/1 -> EtherCAT PDO Transmit 5/1
  velocity override/1 -> EtherCAT PDO Transmit 3/1
  velocity setpoint/1 -> EtherCAT PDO Transmit 4/1
  motor enable1/1 -> EtherCAT PDO Transmit 6/1
  velocity override1/1 -> EtherCAT PDO Transmit 1/1
  velocity setpoint1/1 -> EtherCAT PDO Transmit 2/1

== system MARCH_v1_6/EtherCAT Motor Parameters/Right Leg ==
  EtherCAT PDO Transmit 1 : xpcethercatlib/EtherCAT PDO Transmit   Priority=3  sig_name=Right_Leg.Outputs.K_data[4]  sig_offset=2376  sig_type=int32  type_size=32  sig_dim=1  device_id=0  sample_time=0.001000
  EtherCAT PDO Transmit 2 : xpcethercatlib/EtherCAT PDO Transmit   Priority=3  sig_name=Right_Leg.Outputs.K_velocitySetPoint  sig_offset=2120  sig_type=int16  type_size=16  sig_dim=1  device_id=0  sample_time=0.001000
  EtherCAT PDO Transmit 3 : xpcethercatlib/EtherCAT PDO Transmit   Priority=3  sig_name=Right_Leg.Outputs.H_data[4]  sig_offset=2088  sig_type=int32  type_size=32  sig_dim=1  device_id=0  sample_time=0.001000
  EtherCAT PDO Transmit 4 : xpcethercatlib/EtherCAT PDO Transmit   Priority=3  sig_name=Right_Leg.Outputs.H_velocitySetPoint  sig_offset=1832  sig_type=int16  type_size=16  sig_dim=1  device_id=0  sample_time=0.001000
  EtherCAT PDO Transmit 5 : xpcethercatlib/EtherCAT PDO Transmit   Priority=3  sig_name=Right_Leg.Outputs.H_motorEnable  sig_offset=1880  sig_type=uint8  type_size=8  sig_dim=1  device_id=0  sample_time=0.001000
  EtherCAT PDO Transmit 6 : xpcethercatlib/EtherCAT PDO Transmit   Priority=3  sig_name=Right_Leg.Outputs.K_motorEnable  sig_offset=2168  sig_type=uint8  type_size=8  sig_dim=1  device_id=0  sample_time=0.001000
  motor enable : Constant  Value=0  OutDataTypeStr=uint8
  motor enable1 : Constant  Value=0  OutDataTypeStr=uint8
  velocity override : Constant  Value=0  OutDataTypeStr=int32
  velocity override1 : Constant  Value=0  OutDataTypeStr=int32
  velocity setpoint : Constant  Value=0  OutDataTypeStr=int16
  velocity setpoint1 : Constant  Value=0  OutDataTypeStr=int16
  wires:
  motor enable/1 -> EtherCAT PDO Transmit 5/1
  velocity override/1 -> EtherCAT PDO Transmit 3/1
  velocity setpoint/1 -> EtherCAT PDO Transmit 4/1
  motor enable1/1 -> EtherCAT PDO Transmit 6/1
  velocity override1/1 -> EtherCAT PDO Transmit 1/1
  velocity setpoint1/1 -> EtherCAT PDO Transmit 2/1

== system MARCH_v1_6/Input Device/EtherCAT Input Device ==
  EtherCAT PDO Receive : xpcethercatlib/EtherCAT PDO Receive  Priority=2  sig_name=Hip_HAA.Inputs.L_crutchTrigger  sig_offset=320  sig_type=uint8  type_size=8  sig_dim=1  device_id=0  sample_time=0.001000
  Input Device : Outport
  wires:
  EtherCAT PDO Receive/1 -> Input Device/1

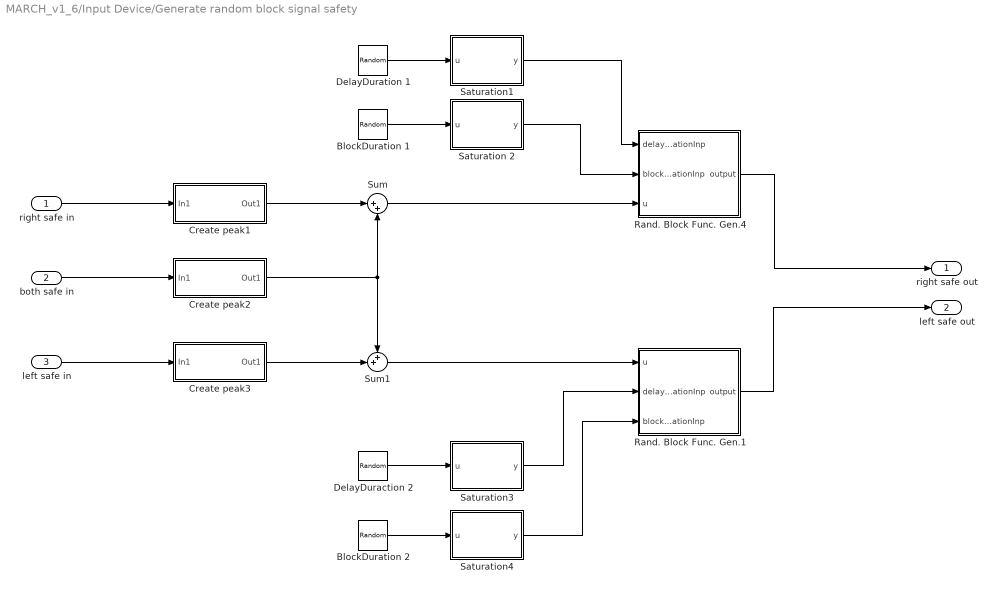
== system MARCH_v1_6/Input Device/Generate random block signal safety ==
  right safe in : Inport
  both safe in : Inport  Port=2
  "left safe in " : Inport  Port=3
  BlockDuration 1 : RandomNumber  Mean=1  Variance=0.1^2  Seed=floor(1000*rand(1,1))  SampleTime=0.001
  BlockDuration 2 : RandomNumber  Mean=1  Variance=0.1^1  Seed=floor(1000*rand(1,1))  SampleTime=0.001
  Create peak1 : Subsystem
  Create peak2 : Subsystem
  Create peak3 : Subsystem
  DelayDuraction 2 : RandomNumber  Mean=0.2  Variance=0.05^2  Seed=floor(1000*rand(1,1))  SampleTime=0.001
  DelayDuration 1 : RandomNumber  Mean=0.2  Variance=0.05^2  Seed=floor(1000*rand(1,1))  SampleTime=0.001
  Rand. Block Func. Gen.1 : MATLAB Function  TreatAsAtomicUnit=on
  Rand. Block Func. Gen.4 : MATLAB Function  TreatAsAtomicUnit=on
  Saturation 2 : MATLAB Function  TreatAsAtomicUnit=on
  Saturation1 : MATLAB Function  TreatAsAtomicUnit=on
  "Saturation3 " : MATLAB Function  TreatAsAtomicUnit=on
  Saturation4 : MATLAB Function  TreatAsAtomicUnit=on
  Sum : Sum  Inputs=|++
  Sum1 : Sum  Inputs=++|
  right safe out : Outport
  left safe out : Outport  Port=2
  wires:
  BlockDuration 2/1 -> Saturation4/1(u)
  DelayDuraction 2/1 -> "Saturation3 "/1(u)
  right safe in/1 -> Create peak1/1(In1)
  Saturation1/1(y) -> Rand. Block Func. Gen.4/1(delayDurationInp)
  Saturation 2/1(y) -> Rand. Block Func. Gen.4/2(blockDurationInp)
  Saturation4/1(y) -> Rand. Block Func. Gen.1/3(blockDurationInp)
  BlockDuration 1/1 -> Saturation 2/1(u)
  DelayDuration 1/1 -> Saturation1/1(u)
  "Saturation3 "/1(y) -> Rand. Block Func. Gen.1/2(delayDurationInp)
  Rand. Block Func. Gen.1/1(output) -> left safe out/1
  Rand. Block Func. Gen.4/1(output) -> right safe out/1
  Create peak1/1(Out1) -> Sum/1
  both safe in/1 -> Create peak2/1(In1)
  "left safe in "/1 -> Create peak3/1(In1)
  Create peak2/1(Out1) -> Sum1/1, Sum/2
  Sum/1 -> Rand. Block Func. Gen.4/3(u)
  Create peak3/1(Out1) -> Sum1/2
  Sum1/1 -> Rand. Block Func. Gen.1/1(u)

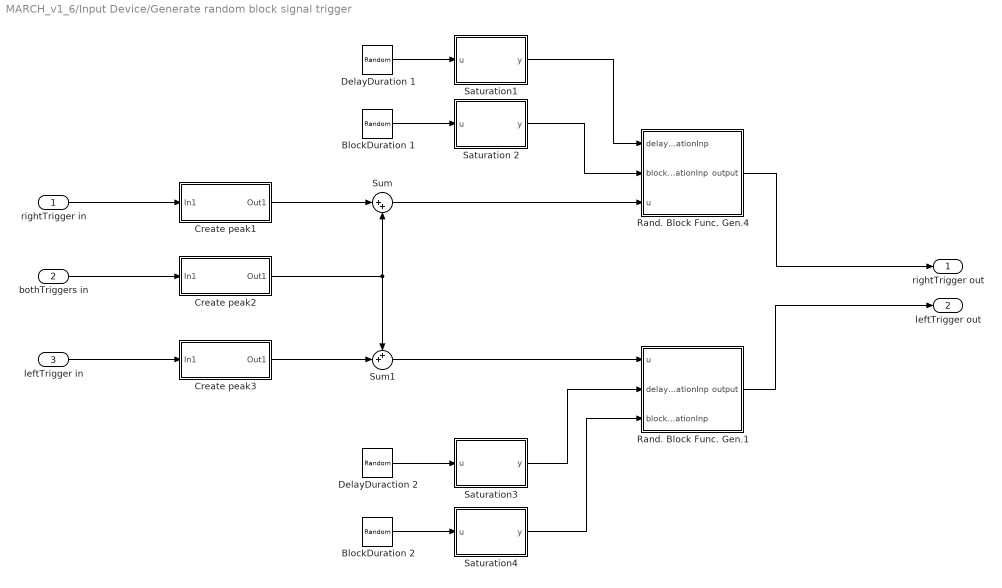
== system MARCH_v1_6/Input Device/Generate random block signal trigger ==
  rightTrigger in : Inport
  bothTriggers in : Inport  Port=2
  "leftTrigger in " : Inport  Port=3
  BlockDuration 1 : RandomNumber  Mean=1  Variance=0.1^2  Seed=floor(1000*rand(1,1))  SampleTime=0.001
  BlockDuration 2 : RandomNumber  Mean=1  Variance=0.1^2  Seed=floor(1000*rand(1,1))  SampleTime=0.001
  Create peak1 : Subsystem
  Create peak2 : Subsystem
  Create peak3 : Subsystem
  DelayDuraction 2 : RandomNumber  Mean=0.2  Variance=0.05^2  Seed=floor(1000*rand(1,1))  SampleTime=0.001
  DelayDuration 1 : RandomNumber  Mean=0.2  Variance=0.05^2  Seed=floor(1000*rand(1,1))  SampleTime=0.001
  Rand. Block Func. Gen.1 : MATLAB Function  TreatAsAtomicUnit=on
  Rand. Block Func. Gen.4 : MATLAB Function  TreatAsAtomicUnit=on
  Saturation 2 : MATLAB Function  TreatAsAtomicUnit=on
  Saturation1 : MATLAB Function  TreatAsAtomicUnit=on
  "Saturation3 " : MATLAB Function  TreatAsAtomicUnit=on
  Saturation4 : MATLAB Function  TreatAsAtomicUnit=on
  Sum : Sum  Inputs=|++
  Sum1 : Sum  Inputs=++|
  rightTrigger out : Outport
  leftTrigger out : Outport  Port=2
  wires:
  BlockDuration 2/1 -> Saturation4/1(u)
  DelayDuraction 2/1 -> "Saturation3 "/1(u)
  rightTrigger in/1 -> Create peak1/1(In1)
  Saturation1/1(y) -> Rand. Block Func. Gen.4/1(delayDurationInp)
  Saturation 2/1(y) -> Rand. Block Func. Gen.4/2(blockDurationInp)
  Saturation4/1(y) -> Rand. Block Func. Gen.1/3(blockDurationInp)
  BlockDuration 1/1 -> Saturation 2/1(u)
  DelayDuration 1/1 -> Saturation1/1(u)
  "Saturation3 "/1(y) -> Rand. Block Func. Gen.1/2(delayDurationInp)
  Rand. Block Func. Gen.1/1(output) -> leftTrigger out/1
  Rand. Block Func. Gen.4/1(output) -> rightTrigger out/1
  Create peak1/1(Out1) -> Sum/1
  bothTriggers in/1 -> Create peak2/1(In1)
  "leftTrigger in "/1 -> Create peak3/1(In1)
  Create peak2/1(Out1) -> Sum1/1, Sum/2
  Sum/1 -> Rand. Block Func. Gen.4/3(u)
  Create peak3/1(Out1) -> Sum1/2
  Sum1/1 -> Rand. Block Func. Gen.1/1(u)

== system MARCH_v1_6/Point&Go/EtherCAT Point&Go ==
  EtherCAT PDO Receive : xpcethercatlib/EtherCAT PDO Receive  Priority=2  sig_name=Hip_HAA.Inputs.R_crutchProximity[0]  sig_offset=984  sig_type=uint32  type_size=32  sig_dim=1  device_id=0  sample_time=0.001000
  Point&Go Data : Outport
  wires:
  EtherCAT PDO Receive/1 -> Point&Go Data/1

== system MARCH_v1_6/State Machine/Create peak3 ==
  In1 : Inport
  Delay : Delay  DelayLength=1
  Greater than 0 : MATLAB Function  TreatAsAtomicUnit=on
  Sum : Sum  Inputs=|-+
  Out1 : Outport
  wires:
  Sum/1 -> Greater than 0/1(peak)
  In1/1 -> Sum/2, Delay/1
  Delay/1 -> Sum/1
  Greater than 0/1(signal) -> Out1/1

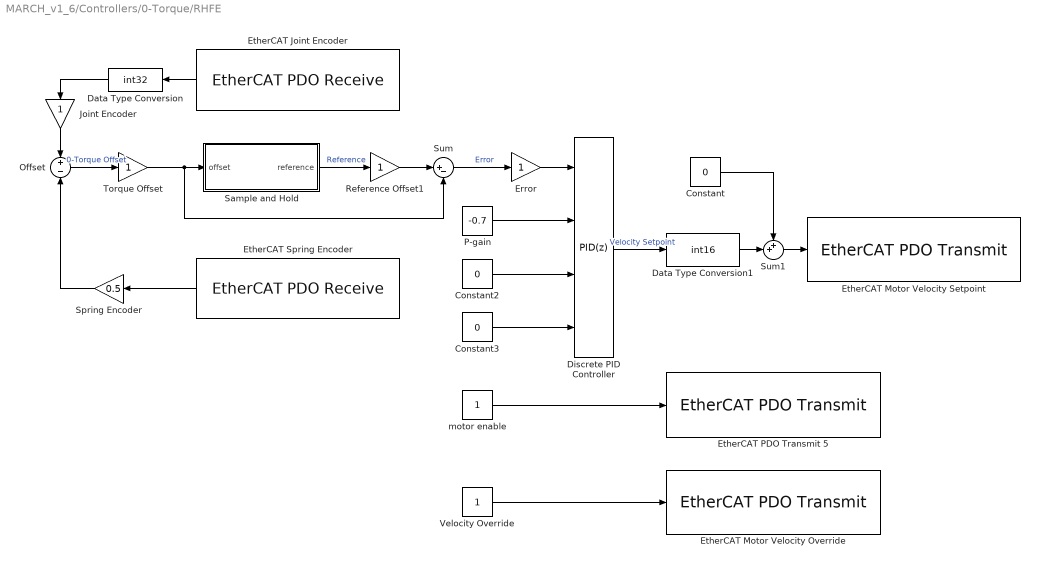
== system MARCH_v1_6/Controllers/0-Torque/RHFE ==
  Constant : Constant  Value=0  OutDataTypeStr=int16
  Constant2 : Constant  Value=0
  Constant3 : Constant  Value=0
  Data Type Conversion : DataTypeConversion  OutDataTypeStr=int32
  Data Type Conversion1 : DataTypeConversion  OutDataTypeStr=int16
  Discrete PID Controller : simulink/Continuous/PID Controller  Controller=PID  TimeDomain=Discrete-time  SampleTime=-1  IntegratorMethod=Forward Euler  FilterMethod=Forward Euler  Form=Parallel  UseFilter=off  ControllerParametersSource=external  P=-0.7  I=0  D=0  N=100  InitialConditionSource=internal  InitialConditionForIntegrator=0  InitialConditionForFilter=0  ExternalReset=none  LimitOutput=on  UpperSaturationLimit=500  LowerSaturationLimit=-500  LinearizeAsGain=off  AntiWindupMode=none  Kb=1  TrackingMode=off  Kt=1  PParamMin=[]  PParamMax=[]  IParamMin=[]  IParamMax=[]  DParamMin=[]  DParamMax=[]  NParamMin=[]  NParamMax=[]  KbParamMin=[]  KbParamMax=[]  KtParamMin=[]  KtParamMax=[]  POutMin=[]  POutMax=[]  IOutMin=[]  IOutMax=[]  DOutMin=[]  DOutMax=[]  NOutMin=[]  NOutMax=[]  KbOutMin=[]  KbOutMax=[]  KtOutMin=[]  KtOutMax=[]  IntegratorOutMin=[]  IntegratorOutMax=[]  FilterOutMin=[]  FilterOutMax=[]  SumOutMin=[]  SumOutMax=[]  SumOutDataTypeStr=int16  SumI1OutMin=[]  SumI1OutMax=[]  SumI2OutMin=[]  SumI2OutMax=[]  SumI3OutMin=[]  SumI3OutMax=[]  SumDOutMin=[]  SumDOutMax=[]  SaturationOutMin=[]  SaturationOutMax=[]  IntegratorContinuousStateAttributes=''  IntegratorStateMustResolveToSignalObject=off  IntegratorRTWStateStorageClass=Auto  FilterContinuousStateAttributes=''  FilterStateMustResolveToSignalObject=off  FilterRTWStateStorageClass=Auto  DifferentiatorICPrevScaledInput=0  DifferentiatorOutMin=[]  DifferentiatorOutMax=[]
  "Error " : Gain  OutDataTypeStr=int32
  EtherCAT Joint Encoder : xpcethercatlib/EtherCAT PDO Receive  Priority=2  sig_name=Right_Leg.Inputs.H_jointAngle  sig_offset=1832  sig_type=uint32  type_size=32  sig_dim=1  device_id=0  sample_time=0.001000
  EtherCAT Motor Velocity Override : xpcethercatlib/EtherCAT PDO Transmit   Priority=3  sig_name=Right_Leg.Outputs.H_data[4]  sig_offset=2088  sig_type=int32  type_size=32  sig_dim=1  device_id=0  sample_time=0.001000
  EtherCAT Motor Velocity Setpoint : xpcethercatlib/EtherCAT PDO Transmit   Priority=3  sig_name=Right_Leg.Outputs.H_velocitySetPoint  sig_offset=1832  sig_type=int16  type_size=16  sig_dim=1  device_id=0  sample_time=0.001000
  EtherCAT PDO Transmit 5 : xpcethercatlib/EtherCAT PDO Transmit   Priority=3  sig_name=Right_Leg.Outputs.H_motorEnable  sig_offset=1880  sig_type=uint8  type_size=8  sig_dim=1  device_id=0  sample_time=0.001000
  EtherCAT Spring Encoder : xpcethercatlib/EtherCAT PDO Receive  Priority=2  sig_name=Right_Leg.Inputs.H_springAngle  sig_offset=1864  sig_type=uint32  type_size=32  sig_dim=1  device_id=0  sample_time=0.001000
  Joint Encoder : Gain  OutDataTypeStr=int32
  Offset : Sum  Inputs=+|-
  P-gain : Constant  Value=-0.7
  Reference Offset1 : Gain  OutDataTypeStr=int32
  Sample and Hold : MATLAB Function  TreatAsAtomicUnit=on
  Spring Encoder : Gain  Gain=0.5  OutDataTypeStr=int32
  Sum : Sum  Inputs=|+-  AccumDataTypeStr=uint32
  Sum1 : Sum  Inputs=++|
  Torque Offset : Gain  OutDataTypeStr=int32
  Velocity Override : Constant  OutDataTypeStr=int32
  motor enable : Constant  OutDataTypeStr=uint8
  wires:
  EtherCAT Joint Encoder/1 -> Data Type Conversion/1
  EtherCAT Spring Encoder/1 -> Spring Encoder/1
  Offset/1 -> Torque Offset/1  "0-Torque Offset"
  Sample and Hold/1(reference) -> Reference Offset1/1  "Reference"
  Sum/1 -> "Error "/1  "Error"
  Velocity Override/1 -> EtherCAT Motor Velocity Override/1
  Spring Encoder/1 -> Offset/2
  Data Type Conversion/1 -> Joint Encoder/1
  Joint Encoder/1 -> Offset/1
  Torque Offset/1 -> Sample and Hold/1(offset), Sum/2
  Reference Offset1/1 -> Sum/1
  "Error "/1 -> Discrete PID Controller/1
  Sum1/1 -> EtherCAT Motor Velocity Setpoint/1
  Discrete PID Controller/1 -> Data Type Conversion1/1  "Velocity Setpoint"
  Constant/1 -> Sum1/1
  motor enable/1 -> EtherCAT PDO Transmit 5/1
  Data Type Conversion1/1 -> Sum1/2
  P-gain/1 -> Discrete PID Controller/2
  Constant2/1 -> Discrete PID Controller/3
  Constant3/1 -> Discrete PID Controller/4

== system MARCH_v1_6/Controllers/Continuous Gait/Slider ==

== system MARCH_v1_6/EtherCAT Joint Setpoints/exoskeleton/EtherCAT Joint Communication ==
  Joint Setpoints : Inport
  Demux : Demux  Outputs=6
  "EtherCAT PDO Transmit " : xpcethercatlib/EtherCAT PDO Transmit   Priority=3  Commented=on  sig_name=LKFE.Outputs.jointSetpoint  sig_offset=496  sig_type=uint32  type_size=32  sig_dim=1  device_id=0  sample_time=0.001000
  EtherCAT PDO Transmit 1 : xpcethercatlib/EtherCAT PDO Transmit   Priority=3  sig_name=RHFE.Outputs.jointSetpoint  sig_offset=12496  sig_type=uint32  type_size=32  sig_dim=1  device_id=0  sample_time=0.001000
  EtherCAT PDO Transmit 2 : xpcethercatlib/EtherCAT PDO Transmit   Priority=3  sig_name=RKFE.Outputs.jointSetpoint  sig_offset=12784  sig_type=uint32  type_size=32  sig_dim=1  device_id=0  sample_time=0.001000
  EtherCAT PDO Transmit 3 : xpcethercatlib/EtherCAT PDO Transmit   Priority=3  Commented=on  sig_name=LHFE.Outputs.data0  sig_offset=240  sig_type=uint32  type_size=32  sig_dim=1  device_id=0  sample_time=0.001000
  EtherCAT PDO Transmit 4 : xpcethercatlib/EtherCAT PDO Transmit   Priority=3  sig_name=LHFE.Outputs.jointSetpoint  sig_offset=208  sig_type=uint32  type_size=32  sig_dim=1  device_id=0  sample_time=0.001000
  EtherCAT PDO Transmit 5 : xpcethercatlib/EtherCAT PDO Transmit   Priority=3  sig_name=LKFE.Outputs.jointSetpoint  sig_offset=496  sig_type=uint32  type_size=32  sig_dim=1  device_id=0  sample_time=0.001000
  wires:
  Demux/5 -> EtherCAT PDO Transmit 4/1
  Demux/6 -> EtherCAT PDO Transmit 5/1
  Demux/4 -> EtherCAT PDO Transmit 3/1
  Demux/1 -> "EtherCAT PDO Transmit "/1
  Demux/2 -> EtherCAT PDO Transmit 1/1
  Joint Setpoints/1 -> Demux/1
  Demux/3 -> EtherCAT PDO Transmit 2/1

== system MARCH_v1_6/Input Device/Generate random block signal safety/Create peak1 ==
  In1 : Inport
  Delay : Delay  DelayLength=1
  Greater than 0 : MATLAB Function  TreatAsAtomicUnit=on
  Sum : Sum  Inputs=|-+
  Out1 : Outport
  wires:
  Sum/1 -> Greater than 0/1(peak)
  In1/1 -> Sum/2, Delay/1
  Delay/1 -> Sum/1
  Greater than 0/1(signal) -> Out1/1
